simulink model "Accel_Data_ETR07"  (R2017b)
settings: Solver=FixedStepAuto  StartTime=0.0  StopTime=10.0  RelTol=1e-3
libraries: dspfdesign x3
settings Model: Creator=cspt  LastModifiedBy=cspt
settings RTWCC: SystemTargetFile=irt.tlc  TemplateMakefile=irt_default_tmf  Description=INTECRIO Real-Time Target
settings STFCustomTargetCC: TargetLangStandard=C99 (ISO)  UtilityFuncGeneration=Shared location  SystemTargetFile=irt.tlc
settings GRTTargetCC: UtilityFuncGeneration=Shared location  ParMdlRefBuildCompliant=off  CompOptLevelCompliant=off  ConcurrentExecutionCompliant=off  CombineOutputUpdateFcns=off  MatFileLogging=off  CPPClassGenCompliant=off  GRTInterface=on  UseToolchainInfoCompliant=off  GenerateASAP2=on

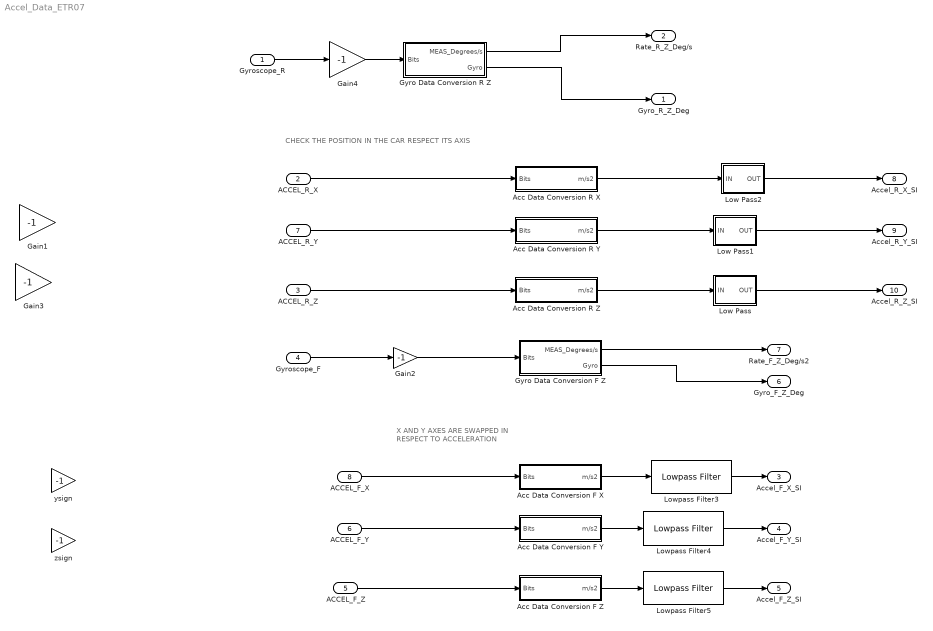
== system Accel_Data_ETR07 ==
  note: CHECK THE POSITION IN THE CAR RESPECT
      | ITS AXIS
  note: X AND Y AXES ARE SWAPPED
      | IN RESPECT TO ACCELERATION
  Gyroscope_R : Inport
  ACCEL_R_X : Inport  Port=2
  ACCEL_R_Z : Inport  Port=3
  Gyroscope_F : Inport  Port=4
  ACCEL_F_Z : Inport  Port=5
  ACCEL_F_Y : Inport  Port=6
  ACCEL_R_Y : Inport  Port=7
  ACCEL_F_X : Inport  Port=8
  Acc Data Conversion F X : Subsystem  TreatAsAtomicUnit=on
  Acc Data Conversion F Y : Subsystem  TreatAsAtomicUnit=on
  Acc Data Conversion F Z : Subsystem  TreatAsAtomicUnit=on
  Acc Data Conversion R X : Subsystem  TreatAsAtomicUnit=on
  Acc Data Conversion R Y : Subsystem  TreatAsAtomicUnit=on
  Acc Data Conversion R Z : Subsystem  TreatAsAtomicUnit=on
  Gain{1..4} (4 alike) : Gain  Gain=-1
  Gyro Data Conversion F Z : Subsystem  TreatAsAtomicUnit=on
  Gyro Data Conversion R Z : Subsystem  TreatAsAtomicUnit=on
  Low Pass : Subsystem  TreatAsAtomicUnit=on
  Low Pass1 : Subsystem  TreatAsAtomicUnit=on
  Low Pass2 : Subsystem  TreatAsAtomicUnit=on
  Lowpass Filter3 : dspfdesign/Lowpass Filter  FilterType=IIR  DesignForMinimumOrder=off  FilterOrder=3  PassbandFrequency=10  StopbandFrequency=1000  PassbandRipple=0.1  StopbandAttenuation=80  InheritSampleRate=on  SampleRate=44100  SimulateUsing=Interpreted execution  roundingMode=Floor  coeffsDataTypeStr=fixdt(1,16)
  Lowpass Filter4 : dspfdesign/Lowpass Filter  FilterType=IIR  DesignForMinimumOrder=off  FilterOrder=3  PassbandFrequency=10  StopbandFrequency=1000  PassbandRipple=0.1  StopbandAttenuation=80  InheritSampleRate=on  SampleRate=44100  SimulateUsing=Interpreted execution  roundingMode=Floor  coeffsDataTypeStr=fixdt(1,16)
  Lowpass Filter5 : dspfdesign/Lowpass Filter  FilterType=IIR  DesignForMinimumOrder=off  FilterOrder=3  PassbandFrequency=10  StopbandFrequency=1000  PassbandRipple=0.1  StopbandAttenuation=80  InheritSampleRate=on  SampleRate=44100  SimulateUsing=Interpreted execution  roundingMode=Floor  coeffsDataTypeStr=fixdt(1,16)
  ysign : Gain  Gain=-1
  zsign : Gain  Gain=-1
  Gyro_R_Z_Deg : Outport
  Rate_R_Z_Deg/s : Outport  Port=2
  Accel_F_X_SI : Outport  Port=3
  Accel_F_Y_SI : Outport  Port=4
  Accel_F_Z_SI : Outport  Port=5
  Gyro_F_Z_Deg : Outport  Port=6
  Rate_F_Z_Deg/s2 : Outport  Port=7
  Accel_R_X_SI : Outport  Port=8
  Accel_R_Y_SI : Outport  Port=9
  Accel_R_Z_SI : Outport  Port=10
  wires:
  Acc Data Conversion F Z/1(m/s2) -> Lowpass Filter5/1
  Acc Data Conversion F Y/1(m/s2) -> Lowpass Filter4/1
  Gyro Data Conversion F Z/1(MEAS_Degrees/s) -> Rate_F_Z_Deg/s2/1
  ACCEL_F_X/1 -> Acc Data Conversion F X/1(Bits)
  Acc Data Conversion F X/1(m/s2) -> Lowpass Filter3/1
  Gyro Data Conversion F Z/2(Gyro) -> Gyro_F_Z_Deg/1
  Gyro Data Conversion R Z/2(Gyro) -> Gyro_R_Z_Deg/1
  ACCEL_R_Z/1 -> Acc Data Conversion R Z/1(Bits)
  Gyro Data Conversion R Z/1(MEAS_Degrees/s) -> Rate_R_Z_Deg/s/1
  Gyroscope_F/1 -> Gain2/1
  Gyroscope_R/1 -> Gain4/1
  Gain4/1 -> Gyro Data Conversion R Z/1(Bits)
  Acc Data Conversion R Y/1(m/s2) -> Low Pass1/1(IN)
  Acc Data Conversion R Z/1(m/s2) -> Low Pass/1(IN)
  Acc Data Conversion R X/1(m/s2) -> Low Pass2/1(IN)
  Gain2/1 -> Gyro Data Conversion F Z/1(Bits)
  ACCEL_R_X/1 -> Acc Data Conversion R X/1(Bits)
  ACCEL_R_Y/1 -> Acc Data Conversion R Y/1(Bits)
  ACCEL_F_Z/1 -> Acc Data Conversion F Z/1(Bits)
  ACCEL_F_Y/1 -> Acc Data Conversion F Y/1(Bits)
  Low Pass2/1(OUT) -> Accel_R_X_SI/1
  Low Pass1/1(OUT) -> Accel_R_Y_SI/1
  Low Pass/1(OUT) -> Accel_R_Z_SI/1
  Lowpass Filter3/1 -> Accel_F_X_SI/1
  Lowpass Filter4/1 -> Accel_F_Y_SI/1
  Lowpass Filter5/1 -> Accel_F_Z_SI/1

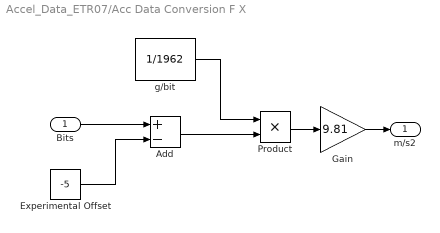
== system Accel_Data_ETR07/Acc Data Conversion F X ==
  Bits : Inport
  Add : Sum  Inputs=+-
  Experimental Offset : Constant  Value=-5
  Gain : Gain  Gain=9.81
  Product : Product
  g/bit : Constant  Value=1/1962
  m/s2 : Outport
  wires:
  Bits/1 -> Add/1
  Experimental Offset/1 -> Add/2
  Add/1 -> Product/2
  g/bit/1 -> Product/1
  Product/1 -> Gain/1
  Gain/1 -> m/s2/1

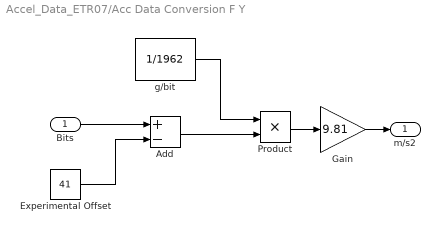
== system Accel_Data_ETR07/Acc Data Conversion F Y ==
  Bits : Inport
  Add : Sum  Inputs=+-
  Experimental Offset : Constant  Value=41
  Gain : Gain  Gain=9.81
  Product : Product
  g/bit : Constant  Value=1/1962
  m/s2 : Outport
  wires:
  Bits/1 -> Add/1
  Experimental Offset/1 -> Add/2
  Add/1 -> Product/2
  g/bit/1 -> Product/1
  Product/1 -> Gain/1
  Gain/1 -> m/s2/1

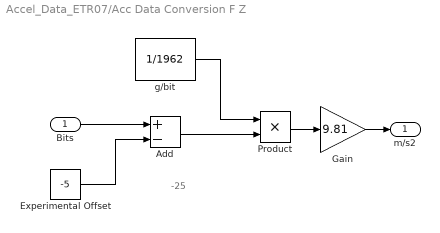
== system Accel_Data_ETR07/Acc Data Conversion F Z ==
  note: -25
  Bits : Inport
  Add : Sum  Inputs=+-
  Experimental Offset : Constant  Value=-5
  Gain : Gain  Gain=9.81
  Product : Product
  g/bit : Constant  Value=1/1962
  m/s2 : Outport
  wires:
  Bits/1 -> Add/1
  Experimental Offset/1 -> Add/2
  Add/1 -> Product/2
  g/bit/1 -> Product/1
  Product/1 -> Gain/1
  Gain/1 -> m/s2/1

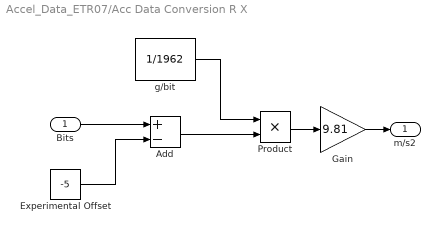
== system Accel_Data_ETR07/Acc Data Conversion R X ==
  Bits : Inport
  Add : Sum  Inputs=+-
  Experimental Offset : Constant  Value=-5
  Gain : Gain  Gain=9.81
  Product : Product
  g/bit : Constant  Value=1/1962
  m/s2 : Outport
  wires:
  Bits/1 -> Add/1
  Experimental Offset/1 -> Add/2
  Add/1 -> Product/2
  g/bit/1 -> Product/1
  Product/1 -> Gain/1
  Gain/1 -> m/s2/1

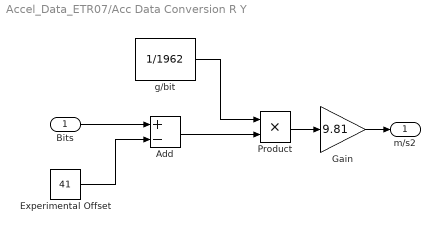
== system Accel_Data_ETR07/Acc Data Conversion R Y ==
  Bits : Inport
  Add : Sum  Inputs=+-
  Experimental Offset : Constant  Value=41
  Gain : Gain  Gain=9.81
  Product : Product
  g/bit : Constant  Value=1/1962
  m/s2 : Outport
  wires:
  Bits/1 -> Add/1
  Experimental Offset/1 -> Add/2
  Add/1 -> Product/2
  g/bit/1 -> Product/1
  Product/1 -> Gain/1
  Gain/1 -> m/s2/1

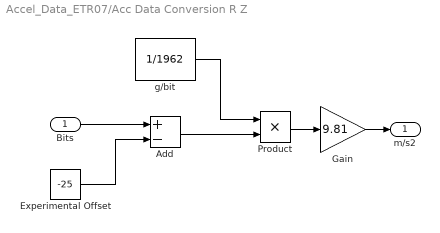
== system Accel_Data_ETR07/Acc Data Conversion R Z ==
  Bits : Inport
  Add : Sum  Inputs=+-
  Experimental Offset : Constant  Value=-25
  Gain : Gain  Gain=9.81
  Product : Product
  g/bit : Constant  Value=1/1962
  m/s2 : Outport
  wires:
  Bits/1 -> Add/1
  Experimental Offset/1 -> Add/2
  Add/1 -> Product/2
  g/bit/1 -> Product/1
  Product/1 -> Gain/1
  Gain/1 -> m/s2/1

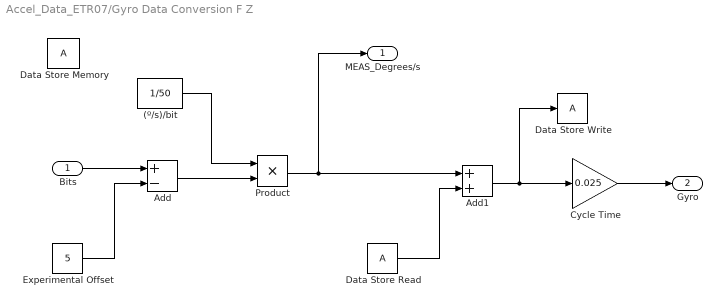
== system Accel_Data_ETR07/Gyro Data Conversion F Z ==
  Bits : Inport
  (º/s)/bit : Constant  Value=1/50
  Add : Sum  Inputs=+-
  Add1 : Sum
  Cycle Time : Gain  Gain=0.025
  Data Store Memory : DataStoreMemory  ReadBeforeWriteMsg=warning  WriteAfterWriteMsg=warning  WriteAfterReadMsg=warning  ShowAdditionalParam=off
  Data Store Read : DataStoreRead
  Data Store Write : DataStoreWrite
  Experimental Offset : Constant  Value=5
  Product : Product
  MEAS_Degrees/s : Outport
  Gyro : Outport  Port=2
  wires:
  Experimental Offset/1 -> Add/2
  Bits/1 -> Add/1
  Add/1 -> Product/2
  (º/s)/bit/1 -> Product/1
  Data Store Read/1 -> Add1/2
  Add1/1 -> Cycle Time/1, Data Store Write/1
  Product/1 -> Add1/1, MEAS_Degrees/s/1
  Cycle Time/1 -> Gyro/1

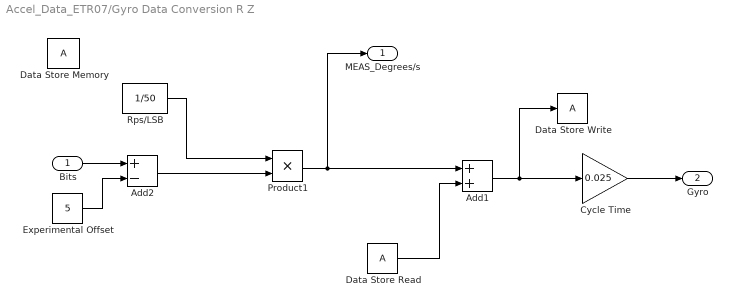
== system Accel_Data_ETR07/Gyro Data Conversion R Z ==
  Bits : Inport
  Add1 : Sum
  Add2 : Sum  Inputs=+-
  Cycle Time : Gain  Gain=0.025
  Data Store Memory : DataStoreMemory  ReadBeforeWriteMsg=warning  WriteAfterWriteMsg=warning  WriteAfterReadMsg=warning  ShowAdditionalParam=off
  Data Store Read : DataStoreRead
  Data Store Write : DataStoreWrite
  Experimental Offset : Constant  Value=5
  Product1 : Product
  Rps/LSB : Constant  Value=1/50
  MEAS_Degrees/s : Outport
  Gyro : Outport  Port=2
  wires:
  Data Store Read/1 -> Add1/2
  Add1/1 -> Cycle Time/1, Data Store Write/1
  Cycle Time/1 -> Gyro/1
  Add2/1 -> Product1/2
  Rps/LSB/1 -> Product1/1
  Product1/1 -> MEAS_Degrees/s/1, Add1/1
  Bits/1 -> Add2/1
  Experimental Offset/1 -> Add2/2

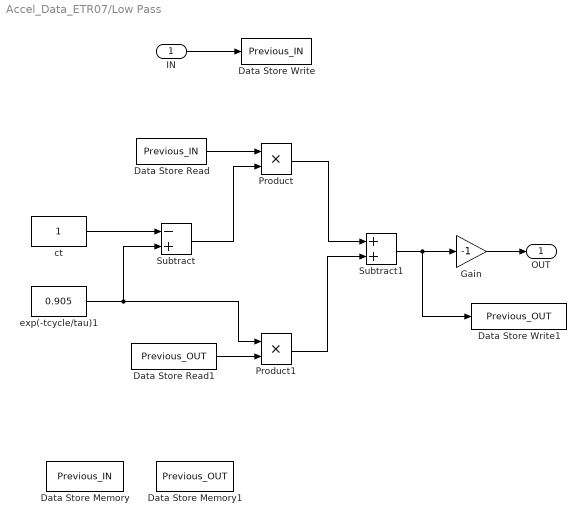
== system Accel_Data_ETR07/Low Pass ==
  IN : Inport
  Data Store Memory : DataStoreMemory  DataStoreName=Previous_IN  ReadBeforeWriteMsg=warning  WriteAfterWriteMsg=warning  WriteAfterReadMsg=warning  ShowAdditionalParam=off
  Data Store Memory1 : DataStoreMemory  DataStoreName=Previous_OUT  ReadBeforeWriteMsg=warning  WriteAfterWriteMsg=warning  WriteAfterReadMsg=warning  ShowAdditionalParam=off
  Data Store Read : DataStoreRead  DataStoreName=Previous_IN
  Data Store Read1 : DataStoreRead  DataStoreName=Previous_OUT
  Data Store Write : DataStoreWrite  DataStoreName=Previous_IN
  Data Store Write1 : DataStoreWrite  DataStoreName=Previous_OUT
  Gain : Gain  Gain=-1
  Product : Product
  Product1 : Product
  Subtract : Sum  Inputs=-+
  Subtract1 : Sum
  ct : Constant
  exp(-tcycle/tau)1 : Constant  Value=0.905
  OUT : Outport
  wires:
  IN/1 -> Data Store Write/1
  Data Store Read/1 -> Product/1
  Data Store Read1/1 -> Product1/2
  ct/1 -> Subtract/1
  Subtract/1 -> Product/2
  exp(-tcycle/tau)1/1 -> Product1/1, Subtract/2
  Product/1 -> Subtract1/1
  Product1/1 -> Subtract1/2
  Subtract1/1 -> Gain/1, Data Store Write1/1
  Gain/1 -> OUT/1

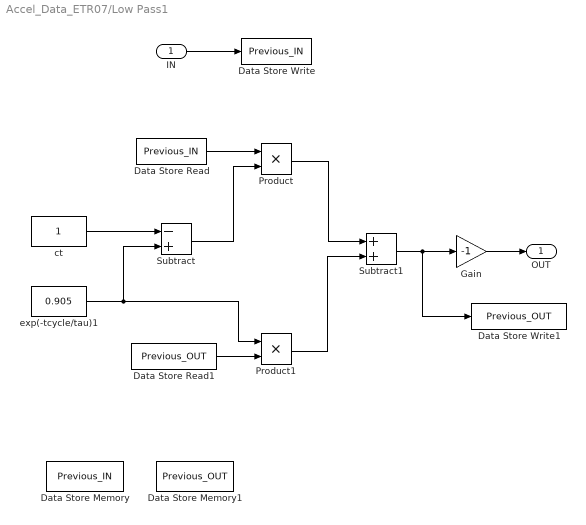
== system Accel_Data_ETR07/Low Pass1 ==
  IN : Inport
  Data Store Memory : DataStoreMemory  DataStoreName=Previous_IN  ReadBeforeWriteMsg=warning  WriteAfterWriteMsg=warning  WriteAfterReadMsg=warning  ShowAdditionalParam=off
  Data Store Memory1 : DataStoreMemory  DataStoreName=Previous_OUT  ReadBeforeWriteMsg=warning  WriteAfterWriteMsg=warning  WriteAfterReadMsg=warning  ShowAdditionalParam=off
  Data Store Read : DataStoreRead  DataStoreName=Previous_IN
  Data Store Read1 : DataStoreRead  DataStoreName=Previous_OUT
  Data Store Write : DataStoreWrite  DataStoreName=Previous_IN
  Data Store Write1 : DataStoreWrite  DataStoreName=Previous_OUT
  Gain : Gain  Gain=-1
  Product : Product
  Product1 : Product
  Subtract : Sum  Inputs=-+
  Subtract1 : Sum
  ct : Constant
  exp(-tcycle/tau)1 : Constant  Value=0.905
  OUT : Outport
  wires:
  Gain/1 -> OUT/1
  Subtract1/1 -> Data Store Write1/1, Gain/1
  Product1/1 -> Subtract1/2
  Product/1 -> Subtract1/1
  exp(-tcycle/tau)1/1 -> Subtract/2, Product1/1
  Subtract/1 -> Product/2
  ct/1 -> Subtract/1
  Data Store Read1/1 -> Product1/2
  Data Store Read/1 -> Product/1
  IN/1 -> Data Store Write/1

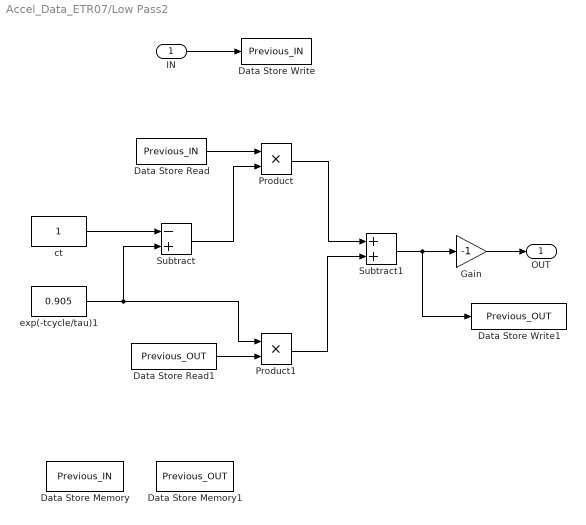
== system Accel_Data_ETR07/Low Pass2 ==
  IN : Inport
  Data Store Memory : DataStoreMemory  DataStoreName=Previous_IN  ReadBeforeWriteMsg=warning  WriteAfterWriteMsg=warning  WriteAfterReadMsg=warning  ShowAdditionalParam=off
  Data Store Memory1 : DataStoreMemory  DataStoreName=Previous_OUT  ReadBeforeWriteMsg=warning  WriteAfterWriteMsg=warning  WriteAfterReadMsg=warning  ShowAdditionalParam=off
  Data Store Read : DataStoreRead  DataStoreName=Previous_IN
  Data Store Read1 : DataStoreRead  DataStoreName=Previous_OUT
  Data Store Write : DataStoreWrite  DataStoreName=Previous_IN
  Data Store Write1 : DataStoreWrite  DataStoreName=Previous_OUT
  Gain : Gain  Gain=-1
  Product : Product
  Product1 : Product
  Subtract : Sum  Inputs=-+
  Subtract1 : Sum
  ct : Constant
  exp(-tcycle/tau)1 : Constant  Value=0.905
  OUT : Outport
  wires:
  IN/1 -> Data Store Write/1
  Data Store Read/1 -> Product/1
  Data Store Read1/1 -> Product1/2
  ct/1 -> Subtract/1
  Subtract/1 -> Product/2
  exp(-tcycle/tau)1/1 -> Product1/1, Subtract/2
  Product/1 -> Subtract1/1
  Product1/1 -> Subtract1/2
  Subtract1/1 -> Gain/1, Data Store Write1/1
  Gain/1 -> OUT/1
